simulink model "SingleInverterSim"  (R2020b)
settings: Solver=FixedStepAuto  StartTime=0.0  StopTime=3  FixedStep=Ts  RelTol=1e-3
values from neighbouring files (symbols this model uses):
  Cf = 0.02/W    (= 6.36619772368e-05)    [CalcSwingDroop.m]    (also in SingleInverterSim_Para.m = 0.02; SingleInverterSim_Para_v2.m = 0.02)
  Lc = 0.01/W    (= 3.18309886184e-05)    [CalcSwingDroop.m]    (also in SingleInverterSim_Para.m = 1e-09; SingleInverterSim_Para_v2.m = 0.01)
  Lf = 0.05/W    (= 0.000159154943092)    [CalcSwingDroop.m]    (also in SingleInverterSim_Para.m = 0.05; SingleInverterSim_Para_v2.m = 0.05)
  m = m*Wbase    (= 15.7079632679)    [CalcSwingDroop.m]    (also in SingleInverterSim_Para.m = 0.05; SingleInverterSim_Para_v2.m = 0.05)
  R_rated_GFL = X_rated_GFL/5    (= 0.08)    [SingleInverterSim_Para.m]
  R_rated_GFM = X_rated_GFM/5    (= 0.06)    [SingleInverterSim_Para.m]
  Sbase = 1    [MainAnalysisImpedanceCircuit.m]    (also in SingleInverterSim_Para.m; SingleInverterSim_Para_v2.m)
  Scale_ki_v = 20    [SingleInverterSim_Para.m]    (also in SingleInverterSim_Para_v2.m)
  Ts = 1/Fs    (= 0.0001)    [SingleInverterSim_Para.m]    (also in SingleInverterSim_Para_v2.m)
  Vbase = 1    [MainAnalysisImpedanceCircuit.m]    (also in SingleInverterSim_Para.m; SingleInverterSim_Para_v2.m)
  w_droop = 0.1*2*pi    (= 0.628318530718)    [SingleInverterSim_Para.m]    (also in SingleInverterSim_Para_v2.m = 62.8318530718)
  w_i_GFL = 250 *2*pi    (= 1570.79632679)    [SingleInverterSim_Para.m]    (also in SingleInverterSim_Para_v2.m = 3141.59265359)
  w_i_GFM = 500*2*pi    (= 3141.59265359)    [SingleInverterSim_Para.m]    (also in SingleInverterSim_Para_v2.m)
  w_pll = 15 *2*pi    (= 94.2477796077)    [SingleInverterSim_Para.m]    (also in SingleInverterSim_Para_v2.m = 62.8318530718)
  w_tau = 1e3 *2*pi    (= 6283.18530718)    [SingleInverterSim_Para.m]    (also in SingleInverterSim_Para_v2.m)
  w_v_GFM = 250 *2*pi    (= 1570.79632679)    [SingleInverterSim_Para.m]    (also in SingleInverterSim_Para_v2.m)
  Wbase = 2*pi*50    (= 314.159265359)    [CalcSwingDroop.m]    (also in MainAnalysisImpedanceCircuit.m; SingleInverterSim_Para.m; SingleInverterSim_Para_v2.m)
  X_rated_GFL = 0.4    [SingleInverterSim_Para.m]
  X_rated_GFM = 0.3    [SingleInverterSim_Para.m]
  Zbase = Vbase/Ibase    (= 1)    [MainAnalysisImpedanceCircuit.m]    (also in SingleInverterSim_Para.m; SingleInverterSim_Para_v2.m)
undefined symbols (not defined in the file or in its folder): DiscIntNeverNeededParam, initial, magnitude
libraries: powerlib x230, SimplexPS x57, SimplexPS_2015a x10, SimplusGT x3
(part 2 of 5)

== system SingleInverterSim/AC Infinite Bus (Voltage Type)5 ==
  note: Model for voltage-type infinite bus.
      |
      | Author(s): Yitong Li
  note: Electrical Circuit
  note: Auxiliary
  Bus Creator : BusCreator  Inputs=7
  Constant : Constant  Value=[vd vq]
  Constant1 : Constant  Value=w
  Constant2 : Constant  Value=theta0
  Constant3 : Constant  Value=2*pi
  Demux : Demux  Outputs=3
  Discrete-Time Integrator : DiscreteIntegrator  IntegratorMethod=Integration: Trapezoidal  InitialConditionSource=external  SampleTime=-1  ICPrevOutput=DiscIntNeverNeededParam  ICPrevScaledInput=DiscIntNeverNeededParam
  Gain1 : Gain  Gain=Vbase
  Gain2 : Gain  Gain=1/Wbase
  Gain3 : Gain  Gain=1/(Sbase/Vbase)
  Math Function1 : Math  Operator=mod  SignedPower=on  SaturateOnIntegerOverflow=on
  Mux : Mux  Inputs=3
  PQ Calculation (dq-Frame) : SimplexPS/PQ Calculation (dq-Frame)  SystemSampleTime=-1  VariantActivationTime=update diagram  Latency=0  AutoFrameSizeCalculation=off
      settings: SourceProductName=Simplex Power Systems
  Ra : powerlib/Elements/Series RLC Branch  LConnTagsString=__new0  RConnTagsString=__new0  BranchType=R  Resistance=R  Inductance=1e-3  SetiL0=off  InitialCurrent=0  Capacitance=1e-6  Setx0=off  InitialVoltage=0  Measurements=None
  Rb : powerlib/Elements/Series RLC Branch  LConnTagsString=__new0  RConnTagsString=__new0  BranchType=R  Resistance=R  Inductance=1e-3  SetiL0=off  InitialCurrent=0  Capacitance=1e-6  Setx0=off  InitialVoltage=0  Measurements=None
  Rc : powerlib/Elements/Series RLC Branch  LConnTagsString=__new0  RConnTagsString=__new0  BranchType=R  Resistance=R  Inductance=1e-3  SetiL0=off  InitialCurrent=0  Capacitance=1e-6  Setx0=off  InitialVoltage=0  Measurements=None
  "abc -> dq (Power-Invariant)" : SimplexPS/abc -> dq (Power-Invariant)  SystemSampleTime=-1  VariantActivationTime=update diagram  Latency=0  AutoFrameSizeCalculation=off
      settings: SourceProductName=Simplex Power Systems
  "dq -> abc (Power-Invariant)" : SimplexPS/dq -> abc (Power-Invariant)  SystemSampleTime=-1  VariantActivationTime=update diagram  Latency=0  AutoFrameSizeCalculation=off
      settings: SourceProductName=Simplex Power Systems
  ia : powerlib/Measurements/Current Measurement  PhasorSimulation=off  OutputType=Complex  PSBequivalent=0
  ib : powerlib/Measurements/Current Measurement  PhasorSimulation=off  OutputType=Complex  PSBequivalent=0
  ic : powerlib/Measurements/Current Measurement  PhasorSimulation=off  OutputType=Complex  PSBequivalent=0
  va : powerlib/Electrical Sources/Controlled Voltage Source  Initialize=on  Source_Type=AC  Amplitude=0  Phase=0  Frequency=0  Measurements=None
  vb : powerlib/Electrical Sources/Controlled Voltage Source  Initialize=on  Source_Type=AC  Amplitude=0  Phase=0  Frequency=0  Measurements=None
  vc : powerlib/Electrical Sources/Controlled Voltage Source  Initialize=on  Source_Type=AC  Amplitude=0  Phase=0  Frequency=0  Measurements=None
  a : PMIOPort  Side=Left
  b : PMIOPort  Port=2  Side=Left
  c : PMIOPort  Port=3  Side=Left
  n : PMIOPort  Port=4  Side=Left
  m : Outport
  wires:
  [v_abc] -> Gain1/1
  Demux/1 -> va/1
  Demux/2 -> vb/1
  Demux/3 -> vc/1
  Math Function1/1 -> "dq -> abc (Power-Invariant)"/2, [theta]
  Constant2/1 -> Discrete-Time Integrator/2
  Constant1/1 -> Discrete-Time Integrator/1, [w]
  "dq -> abc (Power-Invariant)"/1 -> [v_abc]
  Constant3/1 -> Math Function1/2
  Constant/1 -> "dq -> abc (Power-Invariant)"/1, [v_dq]
  Discrete-Time Integrator/1 -> Math Function1/1
  [v_dq] -> Bus Creator/1  "v_dq"
  [i_abc] -> Bus Creator/4  "i_abc"
  [w] -> Gain2/1  "w"
  [v_abc] -> Bus Creator/3  "v_abc"
  Gain2/1 -> Bus Creator/5  "w"
  [i_dq] -> Bus Creator/2  "i_dq"
  Bus Creator/1 -> m/1
  [theta] -> Bus Creator/6  "theta"
  ia/1 -> Mux/1
  ib/1 -> Mux/2
  ic/1 -> Mux/3
  [i_abc] -> "abc -> dq (Power-Invariant)"/1
  [theta] -> "abc -> dq (Power-Invariant)"/2
  "abc -> dq (Power-Invariant)"/1 -> [i_dq]
  Gain1/1 -> Demux/1
  Mux/1 -> Gain3/1
  Gain3/1 -> [i_abc]
  [v_dq] -> PQ Calculation (dq-Frame)/1  "v_dq"
  [i_dq] -> PQ Calculation (dq-Frame)/2  "i_dq"
  PQ Calculation (dq-Frame)/1 -> [pq]
  [pq] -> Bus Creator/7  "pq"
  connections:
  vc/LConn1 -- n/RConn1 -- va/LConn1 -- vb/LConn1
  ia/RConn1 -- va/RConn1
  ib/RConn1 -- vb/RConn1
  ic/RConn1 -- vc/RConn1
  Ra/RConn1 -- ia/LConn1
  Ra/LConn1 -- a/RConn1
  ib/LConn1 -- Rb/RConn1
  Rb/LConn1 -- b/RConn1
  Rc/RConn1 -- ic/LConn1
  Rc/LConn1 -- c/RConn1

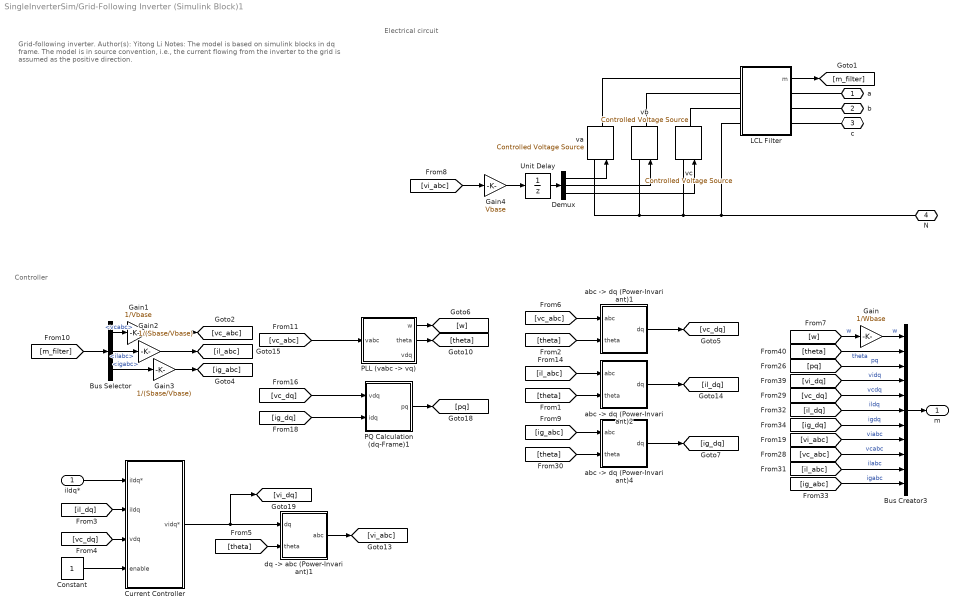
== system SingleInverterSim/Grid-Following Inverter (Simulink Block)1 ==
  note: Grid-following inverter.
      |
      | Author(s): Yitong Li
      |
      | Notes:
      |
      | The model is based on simulink blocks in dq frame.
      |
      | The model is in source convention, i.e., the current flowing from the inverter to the grid is assumed as the positive direction.
  note: Electrical circuit
  note: Controller
  ildq* : Inport
  Bus Creator3 : BusCreator  Inputs=11
  Bus Selector : BusSelector  OutputSignals=vcabc,ilabc,igabc
  Constant : Constant
  Current Controller : Subsystem  mask{Ts=Ts, Wbase=Wbase, Lf=Lf/Wbase, Kg=0, Kp=w_i*Lf/Wbase, Ki=w_i*w_i/4*Lf/Wbase, vdmax=inf, vqmax=inf, Kcd=0}
      mask prompts: Ts "Sampling Time (s)"; Wbase "Base Angular Frequency (rad/s)"; Lf "Inductance"; Kg "Estimator Gain"; Kp "Proportional Gain"; Ki "Integral Gain"; vdmax "Voltage D Limit"; vqmax "Voltage Q Limit"; Kcd "Cross Decoupling Gain"
  Demux : Demux  Outputs=3
  Gain : Gain  Gain=1/Wbase
  Gain1 : Gain  Gain=1/Vbase
  Gain2 : Gain  Gain=1/(Sbase/Vbase)
  Gain3 : Gain  Gain=1/(Sbase/Vbase)
  Gain4 : Gain  Gain=Vbase
  LCL Filter : Subsystem  AncestorBlock=SimplexPS/LCL Filter  mask{Lf=Lf*(Vbase^2/Sbase)/Wbase, Rf=Lf*(Vbase^2/Sbase)/5, Lc=Lc*(Vbase^2/Sbase)/Wbase, Rc=Lc*(Vbase^2/Sbase)/5, Cf=Cf*(Sbase/Vbase^2)/Wbase, Rd=1e-5*(Vbase^2/Sbase)}
      mask prompts: Lf "Lf (H)"; Rf "Rf (Ohm)"; Lc "Lc (H)"; Rc "Rc (Ohm)"; Cf "Cf (F)"; Rd "Rd (Ohm)"
  "PLL (vabc -> vq)" : Subsystem  AncestorBlock=|  mask{Ts=Ts, Vbase=Vbase, Wbase=Wbase, w_pll=w_pll, w_tau=w_tau, theta0=0}
      | SimplusGT/PLL
      | (vabc -> vq)
      mask prompts: Ts "Ts (s), sampling period"; Vbase "Vbase (V), base voltage"; Wbase "Wbase (rad/s), base angular frequency"; w_pll "w_pll (rad/s), PLL bandwidth"; w_tau "w_tau (rad/s), low-pass filter bandwidth"; theta0 "theta0 (rad), initial angle"
  PQ Calculation (dq-Frame)1 : Subsystem  AncestorBlock=|
      | SimplusGT/PQ Calculation
      | (dq-Frame)
  Unit Delay : UnitDelay  SampleTime=-1  HasFrameUpgradeWarning=on
  "abc -> dq (Power-Invariant)1" : Subsystem  AncestorBlock=|
      | SimplusGT/abc -> dq
      | (Power-Invariant)
  "abc -> dq (Power-Invariant)2" : Subsystem  AncestorBlock=|
      | SimplusGT/abc -> dq
      | (Power-Invariant)
  "abc -> dq (Power-Invariant)4" : Subsystem  AncestorBlock=|
      | SimplusGT/abc -> dq
      | (Power-Invariant)
  "dq -> abc (Power-Invariant)1" : Subsystem  AncestorBlock=|
      | SimplusGT/dq -> abc
      | (Power-Invariant)
  va : powerlib/Electrical Sources/Controlled Voltage Source  Initialize=on  Source_Type=AC  Amplitude=0  Phase=0  Frequency=0  Measurements=None
  vb : powerlib/Electrical Sources/Controlled Voltage Source  Initialize=on  Source_Type=AC  Amplitude=0  Phase=0  Frequency=0  Measurements=None
  vc : powerlib/Electrical Sources/Controlled Voltage Source  Initialize=on  Source_Type=AC  Amplitude=0  Phase=0  Frequency=0  Measurements=None
  a : PMIOPort  Side=Right
  b : PMIOPort  Port=2  Side=Right
  c : PMIOPort  Port=3  Side=Right
  N : PMIOPort  Port=4  Side=Right
  m : Outport
  wires:
  [vi_abc] -> Gain4/1
  Gain4/1 -> Unit Delay/1
  Gain3/1 -> [ig_abc]
  Gain2/1 -> [il_abc]
  Gain1/1 -> [vc_abc]
  [ig_abc] -> Bus Creator3/11  "igabc"
  [il_abc] -> Bus Creator3/10  "ilabc"
  [vc_abc] -> Bus Creator3/9  "vcabc"
  [vi_abc] -> Bus Creator3/8  "viabc"
  [ig_dq] -> Bus Creator3/7  "igdq"
  [il_dq] -> Bus Creator3/6  "ildq"
  [vc_dq] -> Bus Creator3/5  "vcdq"
  [vi_dq] -> Bus Creator3/4  "vidq"
  [pq] -> Bus Creator3/3  "pq"
  [theta] -> Bus Creator3/2  "theta"
  Gain/1 -> Bus Creator3/1  "w"
  [w] -> Gain/1  "w"
  Bus Selector/1 -> Gain1/1  "<vcabc>"
  Unit Delay/1 -> Demux/1
  [m_filter] -> Bus Selector/1
  "abc -> dq (Power-Invariant)2"/1(dq) -> [il_dq]
  "abc -> dq (Power-Invariant)4"/1(dq) -> [ig_dq]
  "abc -> dq (Power-Invariant)1"/1(dq) -> [vc_dq]
  [vc_abc] -> "PLL (vabc -> vq)"/1(vabc)
  [il_dq] -> Current Controller/2(iIdq)
  ildq*/1 -> Current Controller/1(iIdq*)
  [ig_dq] -> PQ Calculation (dq-Frame)1/2(idq)
  PQ Calculation (dq-Frame)1/1(pq) -> [pq]
  [vc_dq] -> PQ Calculation (dq-Frame)1/1(vdq)
  [theta] -> "dq -> abc (Power-Invariant)1"/2(theta)
  Current Controller/1(vidq*) -> [vi_dq], "dq -> abc (Power-Invariant)1"/1(dq)
  [vc_dq] -> Current Controller/3(vdq)
  Constant/1 -> Current Controller/4(enable)
  "PLL (vabc -> vq)"/1(w) -> [w]
  "PLL (vabc -> vq)"/2(theta) -> [theta]
  Bus Selector/2 -> Gain2/1  "<ilabc>"
  Bus Selector/3 -> Gain3/1  "<igabc>"
  [theta] -> "abc -> dq (Power-Invariant)4"/2(theta)
  [ig_abc] -> "abc -> dq (Power-Invariant)4"/1(abc)
  [il_abc] -> "abc -> dq (Power-Invariant)2"/1(abc)
  [vc_abc] -> "abc -> dq (Power-Invariant)1"/1(abc)
  [theta] -> "abc -> dq (Power-Invariant)2"/2(theta)
  [theta] -> "abc -> dq (Power-Invariant)1"/2(theta)
  Demux/3 -> vc/1
  Demux/2 -> vb/1
  Demux/1 -> va/1
  LCL Filter/1(m) -> [m_filter]
  Bus Creator3/1 -> m/1
  "dq -> abc (Power-Invariant)1"/1(abc) -> [vi_abc]
  connections:
  LCL Filter/LConn3 -- vc/RConn1
  va/LConn1 -- vb/LConn1 -- vc/LConn1 -- LCL Filter/LConn4 -- N/RConn1
  LCL Filter/RConn3 -- c/RConn1
  LCL Filter/RConn2 -- b/RConn1
  LCL Filter/RConn1 -- a/RConn1
  LCL Filter/LConn1 -- va/RConn1
  LCL Filter/LConn2 -- vb/RConn1

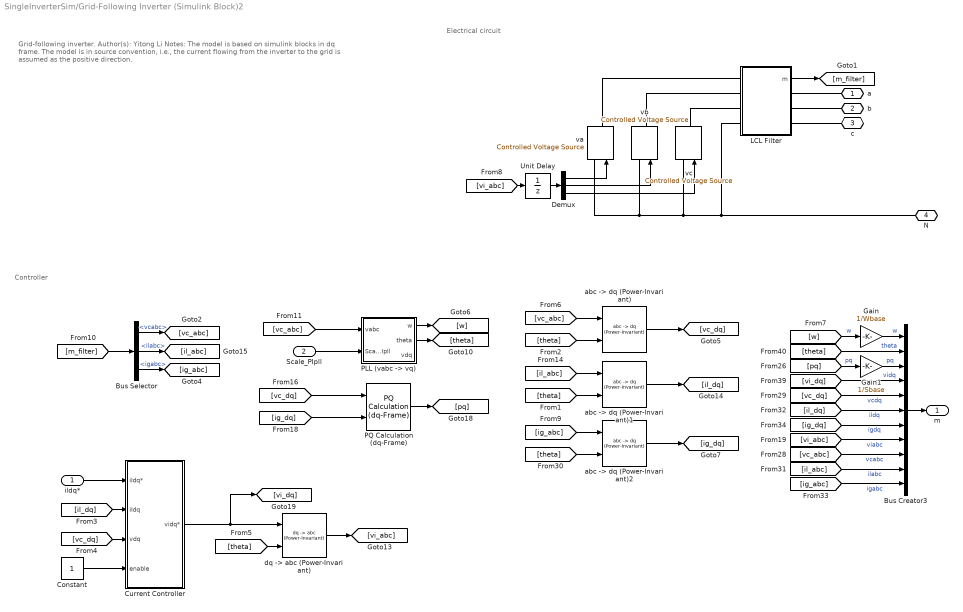
== system SingleInverterSim/Grid-Following Inverter (Simulink Block)2 ==
  note: Controller
  note: Electrical circuit
  note: Grid-following inverter.
      |
      | Author(s): Yitong Li
      |
      | Notes:
      |
      | The model is based on simulink blocks in dq frame.
      |
      | The model is in source convention, i.e., the current flowing from the inverter to the grid is assumed as the positive direction.
  ildq* : Inport
  Scale_PIpll : Inport  Port=2
  Bus Creator3 : BusCreator  Inputs=11
  Bus Selector : BusSelector  OutputSignals=vcabc,ilabc,igabc
  Constant : Constant
  Current Controller : Subsystem  mask{Ts=Ts, Wbase=Wbase, Lf=Lf*(Vbase^2/Sbase)/Wbase, Kg=0, Kp=w_i*Lf*(Vbase^2/Sbase)/Wbase, Ki=w_i*w_i/4*Lf*(Vbase^2/Sbase)/Wbase, vdmax=inf, vqmax=inf, Kcd=0}
      mask prompts: Ts "Sampling Time (s)"; Wbase "Base Angular Frequency (rad/s)"; Lf "Inductance"; Kg "Estimator Gain"; Kp "Proportional Gain"; Ki "Integral Gain"; vdmax "Voltage D Limit"; vqmax "Voltage Q Limit"; Kcd "Cross Decoupling Gain"
  Demux : Demux  Outputs=3
  Gain : Gain  Gain=1/Wbase
  Gain1 : Gain  Gain=1/Sbase
  LCL Filter : Subsystem  AncestorBlock=SimplexPS/LCL Filter  mask{Lf=Lf*Zbase/Wbase, Rf=Lf/5, Lc=Lc*(Vbase^2/Sbase)/Wbase, Rc=Lc/5, Cf=Cf*(Sbase/Vbase^2)/Wbase, Rd=1e-20}
      mask prompts: Lf "Lf (H)"; Rf "Rf (Ohm)"; Lc "Lc (H)"; Rc "Rc (Ohm)"; Cf "Cf (F)"; Rd "Rd (Ohm)"
  "PLL (vabc -> vq)" : Subsystem  AncestorBlock=|  mask{Ts=Ts, Vbase=Vbase, Wbase=Wbase, w_pll=w_pll, w_tau=w_tau, theta0=0}
      | SimplexPS/PLL
      | (vabc -> vq)
      mask prompts: Ts "Ts (s), sampling period"; Vbase "Vbase (V), base voltage"; Wbase "Wbase (rad/s), base angular frequency"; w_pll "w_pll (rad/s), PLL bandwidth"; w_tau "w_tau (rad/s), low-pass filter bandwidth"; theta0 "theta0 (rad), initial angle"
  PQ Calculation (dq-Frame) : SimplexPS/PQ Calculation (dq-Frame)  SystemSampleTime=-1  VariantActivationTime=update diagram  Latency=0  AutoFrameSizeCalculation=off
      settings: SourceProductName=Simplex Power Systems
  Unit Delay : UnitDelay  SampleTime=-1  HasFrameUpgradeWarning=on
  "abc -> dq (Power-Invariant)" : SimplexPS/abc -> dq (Power-Invariant)  SystemSampleTime=-1  VariantActivationTime=update diagram  Latency=0  AutoFrameSizeCalculation=off
      settings: SourceProductName=Simplex Power Systems
  "abc -> dq (Power-Invariant)1" : SimplexPS/abc -> dq (Power-Invariant)  SystemSampleTime=-1  VariantActivationTime=update diagram  Latency=0  AutoFrameSizeCalculation=off
      settings: SourceProductName=Simplex Power Systems
  "abc -> dq (Power-Invariant)2" : SimplexPS/abc -> dq (Power-Invariant)  SystemSampleTime=-1  VariantActivationTime=update diagram  Latency=0  AutoFrameSizeCalculation=off
      settings: SourceProductName=Simplex Power Systems
  "dq -> abc (Power-Invariant)" : SimplexPS/dq -> abc (Power-Invariant)  SystemSampleTime=-1  VariantActivationTime=update diagram  Latency=0  AutoFrameSizeCalculation=off
      settings: SourceProductName=Simplex Power Systems
  va : powerlib/Electrical Sources/Controlled Voltage Source  Initialize=on  Source_Type=AC  Amplitude=0  Phase=0  Frequency=0  Measurements=None
  vb : powerlib/Electrical Sources/Controlled Voltage Source  Initialize=on  Source_Type=AC  Amplitude=0  Phase=0  Frequency=0  Measurements=None
  vc : powerlib/Electrical Sources/Controlled Voltage Source  Initialize=on  Source_Type=AC  Amplitude=0  Phase=0  Frequency=0  Measurements=None
  a : PMIOPort  Side=Right
  b : PMIOPort  Port=2  Side=Right
  c : PMIOPort  Port=3  Side=Right
  N : PMIOPort  Port=4  Side=Right
  m : Outport
  wires:
  "dq -> abc (Power-Invariant)"/1 -> [vi_abc]
  Bus Creator3/1 -> m/1
  LCL Filter/1(m) -> [m_filter]
  Demux/1 -> va/1
  Demux/2 -> vb/1
  Demux/3 -> vc/1
  [theta] -> "abc -> dq (Power-Invariant)"/2
  [theta] -> "abc -> dq (Power-Invariant)1"/2
  [vc_abc] -> "abc -> dq (Power-Invariant)"/1
  [il_abc] -> "abc -> dq (Power-Invariant)1"/1
  [ig_abc] -> "abc -> dq (Power-Invariant)2"/1
  [theta] -> "abc -> dq (Power-Invariant)2"/2
  Bus Selector/3 -> [ig_abc]  "<igabc>"
  Bus Selector/2 -> [il_abc]  "<ilabc>"
  "PLL (vabc -> vq)"/2(theta) -> [theta]
  "PLL (vabc -> vq)"/1(w) -> [w]
  Constant/1 -> Current Controller/4(enable)
  [vc_dq] -> Current Controller/3(vdq)
  Current Controller/1(vidq*) -> [vi_dq], "dq -> abc (Power-Invariant)"/1
  [theta] -> "dq -> abc (Power-Invariant)"/2
  [vc_dq] -> PQ Calculation (dq-Frame)/1
  PQ Calculation (dq-Frame)/1 -> [pq]
  [ig_dq] -> PQ Calculation (dq-Frame)/2
  ildq*/1 -> Current Controller/1(iIdq*)
  [il_dq] -> Current Controller/2(iIdq)
  [vc_abc] -> "PLL (vabc -> vq)"/1(vabc)
  "abc -> dq (Power-Invariant)"/1 -> [vc_dq]
  "abc -> dq (Power-Invariant)2"/1 -> [ig_dq]
  "abc -> dq (Power-Invariant)1"/1 -> [il_dq]
  [m_filter] -> Bus Selector/1
  [vi_abc] -> Unit Delay/1
  Unit Delay/1 -> Demux/1
  Bus Selector/1 -> [vc_abc]  "<vcabc>"
  [w] -> Gain/1  "w"
  [pq] -> Gain1/1  "pq"
  Gain/1 -> Bus Creator3/1  "w"
  [theta] -> Bus Creator3/2  "theta"
  Gain1/1 -> Bus Creator3/3  "pq"
  [vi_dq] -> Bus Creator3/4  "vidq"
  [vc_dq] -> Bus Creator3/5  "vcdq"
  [il_dq] -> Bus Creator3/6  "ildq"
  [ig_dq] -> Bus Creator3/7  "igdq"
  [vi_abc] -> Bus Creator3/8  "viabc"
  [vc_abc] -> Bus Creator3/9  "vcabc"
  [il_abc] -> Bus Creator3/10  "ilabc"
  [ig_abc] -> Bus Creator3/11  "igabc"
  Scale_PIpll/1 -> "PLL (vabc -> vq)"/2(Scale_PIpll)
  connections:
  LCL Filter/LConn2 -- vb/RConn1
  LCL Filter/LConn1 -- va/RConn1
  LCL Filter/RConn1 -- a/RConn1
  LCL Filter/RConn2 -- b/RConn1
  LCL Filter/RConn3 -- c/RConn1
  N/RConn1 -- LCL Filter/LConn4 -- vc/LConn1 -- vb/LConn1 -- va/LConn1
  LCL Filter/LConn3 -- vc/RConn1

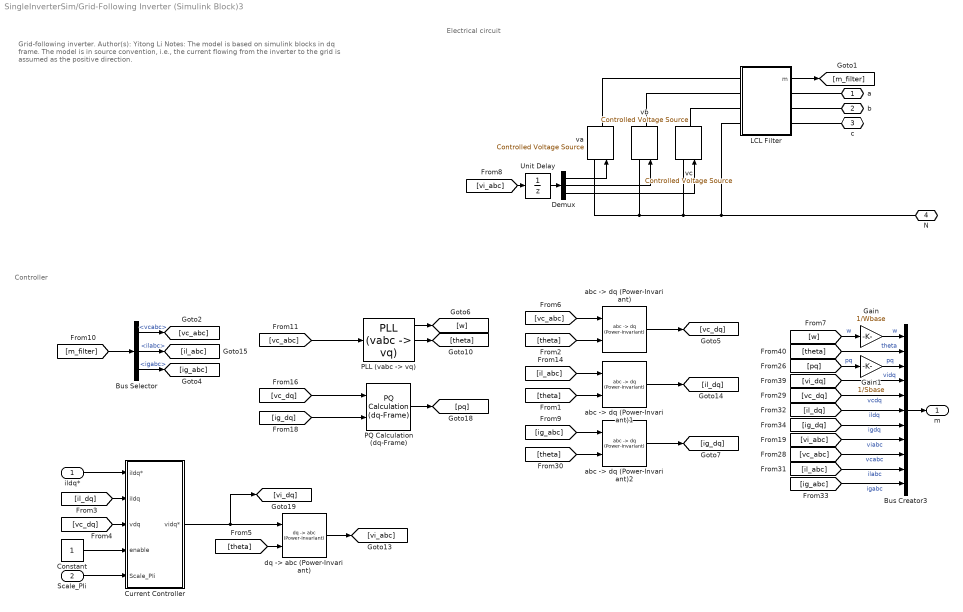
== system SingleInverterSim/Grid-Following Inverter (Simulink Block)3 ==
  note: Controller
  note: Electrical circuit
  note: Grid-following inverter.
      |
      | Author(s): Yitong Li
      |
      | Notes:
      |
      | The model is based on simulink blocks in dq frame.
      |
      | The model is in source convention, i.e., the current flowing from the inverter to the grid is assumed as the positive direction.
  ildq* : Inport
  Scale_PIi : Inport  Port=2
  Bus Creator3 : BusCreator  Inputs=11
  Bus Selector : BusSelector  OutputSignals=vcabc,ilabc,igabc
  Constant : Constant
  Current Controller : Subsystem  mask{Ts=Ts, Wbase=Wbase, Lf=Lf*(Vbase^2/Sbase)/Wbase, Kg=0, Kp=w_i*Lf*(Vbase^2/Sbase)/Wbase, Ki=w_i*w_i/4*Lf*(Vbase^2/Sbase)/Wbase, vdmax=inf, vqmax=inf, Kcd=0}
      mask prompts: Ts "Sampling Time (s)"; Wbase "Base Angular Frequency (rad/s)"; Lf "Inductance"; Kg "Estimator Gain"; Kp "Proportional Gain"; Ki "Integral Gain"; vdmax "Voltage D Limit"; vqmax "Voltage Q Limit"; Kcd "Cross Decoupling Gain"
  Demux : Demux  Outputs=3
  Gain : Gain  Gain=1/Wbase
  Gain1 : Gain  Gain=1/Sbase
  LCL Filter : Subsystem  AncestorBlock=SimplexPS/LCL Filter  mask{Lf=Lf*Zbase/Wbase, Rf=Lf/5, Lc=Lc*(Vbase^2/Sbase)/Wbase, Rc=Lc/5, Cf=Cf*(Sbase/Vbase^2)/Wbase, Rd=1e-20}
      mask prompts: Lf "Lf (H)"; Rf "Rf (Ohm)"; Lc "Lc (H)"; Rc "Rc (Ohm)"; Cf "Cf (F)"; Rd "Rd (Ohm)"
  "PLL (vabc -> vq)" : SimplexPS/PLL (vabc -> vq)  Ts=Ts  Vbase=Vbase  Wbase=Wbase  w_pll=w_pll  w_tau=w_tau  theta0=0
      settings: SourceProductName=Simplex Power Systems
  PQ Calculation (dq-Frame) : SimplexPS/PQ Calculation (dq-Frame)  SystemSampleTime=-1  VariantActivationTime=update diagram  Latency=0  AutoFrameSizeCalculation=off
      settings: SourceProductName=Simplex Power Systems
  Unit Delay : UnitDelay  SampleTime=-1  HasFrameUpgradeWarning=on
  "abc -> dq (Power-Invariant)" : SimplexPS/abc -> dq (Power-Invariant)  SystemSampleTime=-1  VariantActivationTime=update diagram  Latency=0  AutoFrameSizeCalculation=off
      settings: SourceProductName=Simplex Power Systems
  "abc -> dq (Power-Invariant)1" : SimplexPS/abc -> dq (Power-Invariant)  SystemSampleTime=-1  VariantActivationTime=update diagram  Latency=0  AutoFrameSizeCalculation=off
      settings: SourceProductName=Simplex Power Systems
  "abc -> dq (Power-Invariant)2" : SimplexPS/abc -> dq (Power-Invariant)  SystemSampleTime=-1  VariantActivationTime=update diagram  Latency=0  AutoFrameSizeCalculation=off
      settings: SourceProductName=Simplex Power Systems
  "dq -> abc (Power-Invariant)" : SimplexPS/dq -> abc (Power-Invariant)  SystemSampleTime=-1  VariantActivationTime=update diagram  Latency=0  AutoFrameSizeCalculation=off
      settings: SourceProductName=Simplex Power Systems
  va : powerlib/Electrical Sources/Controlled Voltage Source  Initialize=on  Source_Type=AC  Amplitude=0  Phase=0  Frequency=0  Measurements=None
  vb : powerlib/Electrical Sources/Controlled Voltage Source  Initialize=on  Source_Type=AC  Amplitude=0  Phase=0  Frequency=0  Measurements=None
  vc : powerlib/Electrical Sources/Controlled Voltage Source  Initialize=on  Source_Type=AC  Amplitude=0  Phase=0  Frequency=0  Measurements=None
  a : PMIOPort  Side=Right
  b : PMIOPort  Port=2  Side=Right
  c : PMIOPort  Port=3  Side=Right
  N : PMIOPort  Port=4  Side=Right
  m : Outport
  wires:
  "dq -> abc (Power-Invariant)"/1 -> [vi_abc]
  Bus Creator3/1 -> m/1
  LCL Filter/1(m) -> [m_filter]
  Demux/1 -> va/1
  Demux/2 -> vb/1
  Demux/3 -> vc/1
  [theta] -> "abc -> dq (Power-Invariant)"/2
  [theta] -> "abc -> dq (Power-Invariant)1"/2
  [vc_abc] -> "abc -> dq (Power-Invariant)"/1
  [il_abc] -> "abc -> dq (Power-Invariant)1"/1
  [ig_abc] -> "abc -> dq (Power-Invariant)2"/1
  [theta] -> "abc -> dq (Power-Invariant)2"/2
  Bus Selector/3 -> [ig_abc]  "<igabc>"
  Bus Selector/2 -> [il_abc]  "<ilabc>"
  "PLL (vabc -> vq)"/2 -> [theta]
  "PLL (vabc -> vq)"/1 -> [w]
  Constant/1 -> Current Controller/4(enable)
  [vc_dq] -> Current Controller/3(vdq)
  Current Controller/1(vidq*) -> [vi_dq], "dq -> abc (Power-Invariant)"/1
  [theta] -> "dq -> abc (Power-Invariant)"/2
  [vc_dq] -> PQ Calculation (dq-Frame)/1
  PQ Calculation (dq-Frame)/1 -> [pq]
  [ig_dq] -> PQ Calculation (dq-Frame)/2
  ildq*/1 -> Current Controller/1(iIdq*)
  [il_dq] -> Current Controller/2(iIdq)
  [vc_abc] -> "PLL (vabc -> vq)"/1
  "abc -> dq (Power-Invariant)"/1 -> [vc_dq]
  "abc -> dq (Power-Invariant)2"/1 -> [ig_dq]
  "abc -> dq (Power-Invariant)1"/1 -> [il_dq]
  [m_filter] -> Bus Selector/1
  [vi_abc] -> Unit Delay/1
  Unit Delay/1 -> Demux/1
  Bus Selector/1 -> [vc_abc]  "<vcabc>"
  [w] -> Gain/1  "w"
  [pq] -> Gain1/1  "pq"
  Gain/1 -> Bus Creator3/1  "w"
  [theta] -> Bus Creator3/2  "theta"
  Gain1/1 -> Bus Creator3/3  "pq"
  [vi_dq] -> Bus Creator3/4  "vidq"
  [vc_dq] -> Bus Creator3/5  "vcdq"
  [il_dq] -> Bus Creator3/6  "ildq"
  [ig_dq] -> Bus Creator3/7  "igdq"
  [vi_abc] -> Bus Creator3/8  "viabc"
  [vc_abc] -> Bus Creator3/9  "vcabc"
  [il_abc] -> Bus Creator3/10  "ilabc"
  [ig_abc] -> Bus Creator3/11  "igabc"
  Scale_PIi/1 -> Current Controller/5(Scale_PIi)
  connections:
  LCL Filter/LConn2 -- vb/RConn1
  LCL Filter/LConn1 -- va/RConn1
  LCL Filter/RConn1 -- a/RConn1
  LCL Filter/RConn2 -- b/RConn1
  LCL Filter/RConn3 -- c/RConn1
  N/RConn1 -- LCL Filter/LConn4 -- vc/LConn1 -- vb/LConn1 -- va/LConn1
  LCL Filter/LConn3 -- vc/RConn1

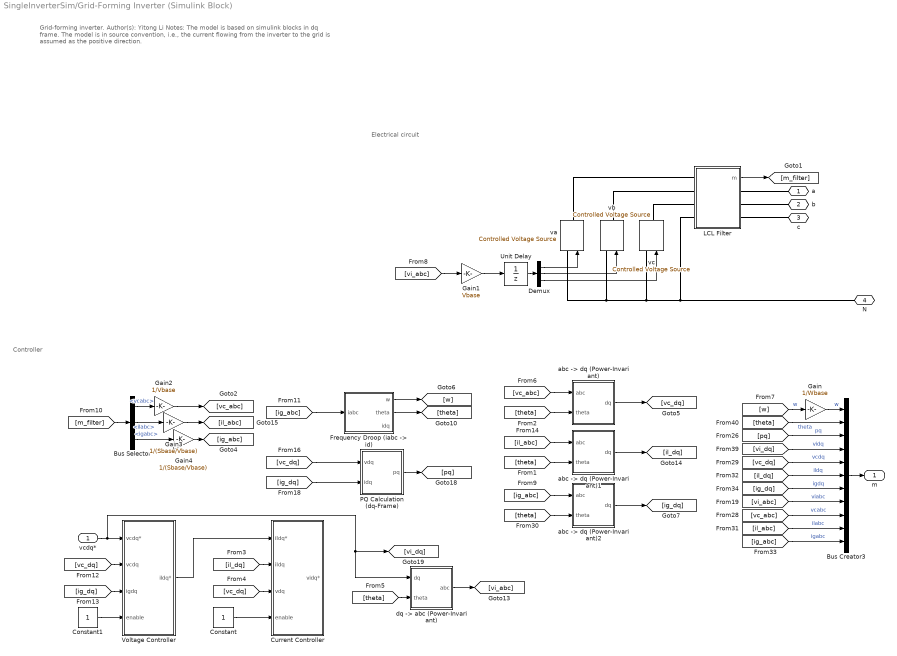
== system SingleInverterSim/Grid-Forming Inverter (Simulink Block) ==
  note: Grid-forming inverter.
      |
      | Author(s): Yitong Li
      |
      | Notes:
      |
      | The model is based on simulink blocks in dq frame.
      |
      | The model is in source convention, i.e., the current flowing from the inverter to the grid is assumed as the positive direction.
  note: Electrical circuit
  note: Controller
  vcdq* : Inport
  Bus Creator3 : BusCreator  Inputs=11
  Bus Selector : BusSelector  OutputSignals=vcabc,ilabc,igabc
  Constant : Constant
  Constant1 : Constant
  Current Controller : Subsystem  mask{Ts=Ts, Wbase=Wbase, Lf=Lf/Wbase, Kg=0, Kp=w_i*Lf/Wbase, Ki=w_i*w_i/4*Lf/Wbase, xdmax=inf, xqmax=inf, Kcd=0}
      mask prompts: Ts "Sampling Time (s)"; Wbase "Base Angular Frequency (rad/s)"; Lf "Inductance"; Kg "Estimator Gain"; Kp "Proportional Gain"; Ki "Integral Gain"; xdmax "Voltage D Limit"; xqmax "Voltage Q Limit"; Kcd "Cross Decoupling Gain"
  Demux : Demux  Outputs=3
  "Frequency Droop (iabc -> id)" : Subsystem  AncestorBlock=|  mask{Ts=Ts, Sbase=Sbase, Vbase=Vbase, Wbase=Wbase, m=m, w_tau=w_droop, theta0=0, i0=0, w0=1}
      | SimplusGT/Frequency Droop
      | (iabc -> id)
      mask prompts: Ts "Ts (s), samping period"; Sbase "Sbase (VA), base power"; Vbase "Vbase (V), base voltage"; Wbase "Wbase (rad/s), base angular frequency"; m "m (pu), droop gain"; w_tau "w_tau (rad/s), low-pass filter bandwidth"; theta0 "theta0 (rad), initial angle"; i0 "i0 (pu), current setting point"; w0 "w0 (pu), frequency setting point"
  Gain : Gain  Gain=1/Wbase
  Gain1 : Gain  Gain=Vbase
  Gain2 : Gain  Gain=1/Vbase
  Gain3 : Gain  Gain=1/(Sbase/Vbase)
  Gain4 : Gain  Gain=1/(Sbase/Vbase)
  LCL Filter : Subsystem  AncestorBlock=SimplexPS/LCL Filter  mask{Lf=Lf*(Vbase^2/Sbase)/Wbase, Rf=Lf*(Vbase^2/Sbase)/5, Lc=Lc*(Vbase^2/Sbase)/Wbase, Rc=Lc*(Vbase^2/Sbase)/5, Cf=Cf*(Sbase/Vbase^2)/Wbase, Rd=1e-5*(Vbase^2/Sbase)}
      mask prompts: Lf "Lf (H)"; Rf "Rf (Ohm)"; Lc "Lc (H)"; Rc "Rc (Ohm)"; Cf "Cf (F)"; Rd "Rd (Ohm)"
  PQ Calculation (dq-Frame) : Subsystem  AncestorBlock=|
      | SimplusGT/PQ Calculation
      | (dq-Frame)
  Unit Delay : UnitDelay  SampleTime=-1  HasFrameUpgradeWarning=on
  Voltage Controller : Subsystem  mask{Ts=Ts, Wbase=Wbase, Cf=Cf/Wbase, Kg=0, Kp=w_v*Cf/Wbase, Ki=w_v*w_v/4*Cf/Wbase*100, xdmax=inf, xqmax=inf, Kcd=0}
      mask prompts: Ts "Sampling Time (s)"; Wbase "Base Angular Frequency (rad/s)"; Cf "Capacitance"; Kg "Estimator Gain"; Kp "Proportional Gain"; Ki "Integral Gain"; xdmax "Current D Limit"; xqmax "Current Q Limit"; Kcd "Cross Decoupling Gain"
  "abc -> dq (Power-Invariant)" : Subsystem  AncestorBlock=|
      | SimplusGT/abc -> dq
      | (Power-Invariant)
  "abc -> dq (Power-Invariant)1" : Subsystem  AncestorBlock=|
      | SimplusGT/abc -> dq
      | (Power-Invariant)
  "abc -> dq (Power-Invariant)2" : Subsystem  AncestorBlock=|
      | SimplusGT/abc -> dq
      | (Power-Invariant)
  "dq -> abc (Power-Invariant)" : Subsystem  AncestorBlock=|
      | SimplusGT/dq -> abc
      | (Power-Invariant)
  va : powerlib/Electrical Sources/Controlled Voltage Source  Initialize=on  Source_Type=AC  Amplitude=0  Phase=0  Frequency=0  Measurements=None
  vb : powerlib/Electrical Sources/Controlled Voltage Source  Initialize=on  Source_Type=AC  Amplitude=0  Phase=0  Frequency=0  Measurements=None
  vc : powerlib/Electrical Sources/Controlled Voltage Source  Initialize=on  Source_Type=AC  Amplitude=0  Phase=0  Frequency=0  Measurements=None
  a : PMIOPort  Side=Right
  b : PMIOPort  Port=2  Side=Right
  c : PMIOPort  Port=3  Side=Right
  N : PMIOPort  Port=4  Side=Right
  m : Outport
  wires:
  Gain1/1 -> Unit Delay/1
  [vi_abc] -> Gain1/1
  Gain4/1 -> [ig_abc]
  Gain3/1 -> [il_abc]
  Gain2/1 -> [vc_abc]
  [ig_dq] -> Voltage Controller/3(igdq)
  [vc_dq] -> Voltage Controller/2(vcdq)
  Constant1/1 -> Voltage Controller/4(enable)
  Voltage Controller/1(ildq*) -> Current Controller/1(iIdq*)
  vcdq*/1 -> [vi_dq], "dq -> abc (Power-Invariant)"/1(dq), Voltage Controller/1(vcdq*)
  [ig_abc] -> Bus Creator3/11  "igabc"
  [il_abc] -> Bus Creator3/10  "ilabc"
  [vc_abc] -> Bus Creator3/9  "vcabc"
  [vi_abc] -> Bus Creator3/8  "viabc"
  [ig_dq] -> Bus Creator3/7  "igdq"
  [il_dq] -> Bus Creator3/6  "ildq"
  [vc_dq] -> Bus Creator3/5  "vcdq"
  [vi_dq] -> Bus Creator3/4  "vidq"
  [pq] -> Bus Creator3/3  "pq"
  [theta] -> Bus Creator3/2  "theta"
  Gain/1 -> Bus Creator3/1  "w"
  [w] -> Gain/1  "w"
  Bus Selector/1 -> Gain2/1  "<vcabc>"
  Unit Delay/1 -> Demux/1
  [m_filter] -> Bus Selector/1
  "abc -> dq (Power-Invariant)1"/1(dq) -> [il_dq]
  "abc -> dq (Power-Invariant)2"/1(dq) -> [ig_dq]
  "abc -> dq (Power-Invariant)"/1(dq) -> [vc_dq]
  [ig_abc] -> "Frequency Droop (iabc -> id)"/1(iabc)
  [il_dq] -> Current Controller/2(iIdq)
  [ig_dq] -> PQ Calculation (dq-Frame)/2(idq)
  PQ Calculation (dq-Frame)/1(pq) -> [pq]
  [vc_dq] -> PQ Calculation (dq-Frame)/1(vdq)
  [theta] -> "dq -> abc (Power-Invariant)"/2(theta)
  [vc_dq] -> Current Controller/3(vdq)
  Constant/1 -> Current Controller/4(enable)
  Bus Selector/2 -> Gain3/1  "<ilabc>"
  Bus Selector/3 -> Gain4/1  "<igabc>"
  [theta] -> "abc -> dq (Power-Invariant)2"/2(theta)
  [ig_abc] -> "abc -> dq (Power-Invariant)2"/1(abc)
  [il_abc] -> "abc -> dq (Power-Invariant)1"/1(abc)
  [vc_abc] -> "abc -> dq (Power-Invariant)"/1(abc)
  [theta] -> "abc -> dq (Power-Invariant)1"/2(theta)
  [theta] -> "abc -> dq (Power-Invariant)"/2(theta)
  Demux/3 -> vc/1
  Demux/2 -> vb/1
  Demux/1 -> va/1
  LCL Filter/1(m) -> [m_filter]
  Bus Creator3/1 -> m/1
  "dq -> abc (Power-Invariant)"/1(abc) -> [vi_abc]
  "Frequency Droop (iabc -> id)"/1(w) -> [w]
  "Frequency Droop (iabc -> id)"/2(theta) -> [theta]
  connections:
  LCL Filter/LConn3 -- vc/RConn1
  va/LConn1 -- vb/LConn1 -- vc/LConn1 -- LCL Filter/LConn4 -- N/RConn1
  LCL Filter/RConn3 -- c/RConn1
  LCL Filter/RConn2 -- b/RConn1
  LCL Filter/RConn1 -- a/RConn1
  LCL Filter/LConn1 -- va/RConn1
  LCL Filter/LConn2 -- vb/RConn1

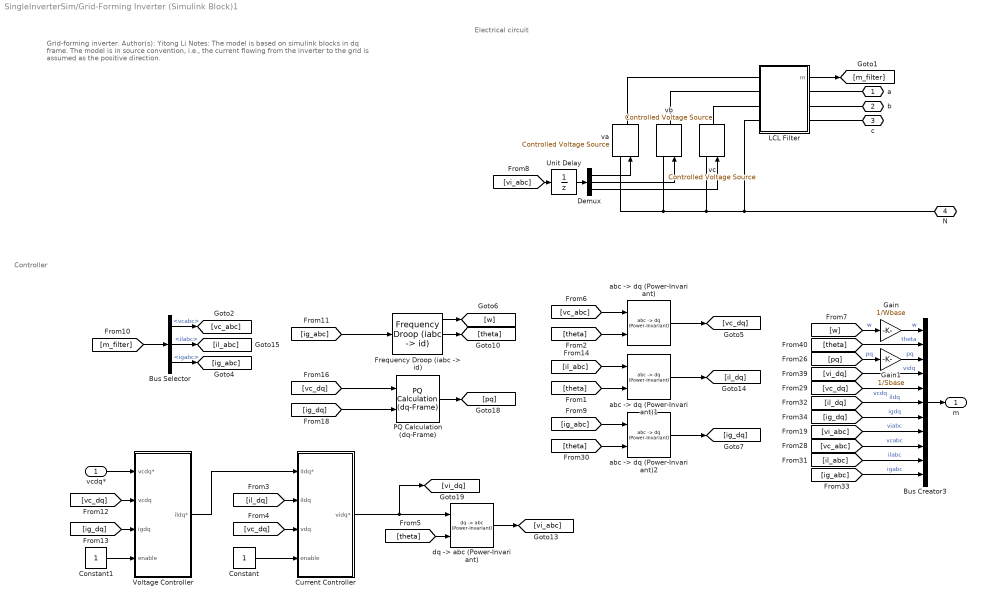
== system SingleInverterSim/Grid-Forming Inverter (Simulink Block)1 ==
  note: Grid-forming inverter.
      |
      | Author(s): Yitong Li
      |
      | Notes:
      |
      | The model is based on simulink blocks in dq frame.
      |
      | The model is in source convention, i.e., the current flowing from the inverter to the grid is assumed as the positive direction.
  note: Electrical circuit
  note: Controller
  vcdq* : Inport
  Bus Creator3 : BusCreator  Inputs=11
  Bus Selector : BusSelector  OutputSignals=vcabc,ilabc,igabc
  Constant : Constant
  Constant1 : Constant
  Current Controller : Subsystem  mask{Ts=Ts, Wbase=Wbase, Lf=Lf*(Vbase^2/Sbase)/Wbase, Kg=0, Kp=w_i*Lf*(Vbase^2/Sbase)/Wbase, Ki=w_i*w_i/4*Lf*(Vbase^2/Sbase)/Wbase, xdmax=inf, xqmax=inf, Kcd=0}
      mask prompts: Ts "Sampling Time (s)"; Wbase "Base Angular Frequency (rad/s)"; Lf "Inductance"; Kg "Estimator Gain"; Kp "Proportional Gain"; Ki "Integral Gain"; xdmax "Voltage D Limit"; xqmax "Voltage Q Limit"; Kcd "Cross Decoupling Gain"
  Demux : Demux  Outputs=3
  "Frequency Droop (iabc -> id)" : SimplexPS/Frequency Droop (iabc -> id)  Ts=Ts  Sbase=Sbase  Vbase=Vbase  Wbase=Wbase  m=m  w_tau=w_droop  theta0=0  i0=0  w0=1
  Gain : Gain  Gain=1/Wbase
  Gain1 : Gain  Gain=1/Sbase
  LCL Filter : Subsystem  AncestorBlock=SimplexPS/LCL Filter  mask{Lf=Lf*(Vbase^2/Sbase)/Wbase, Rf=Lf/10, Lc=Lc*(Vbase^2/Sbase)/Wbase, Rc=1e-20, Cf=Cf*(Sbase/Vbase^2)/Wbase, Rd=1e-20}
      mask prompts: Lf "Lf (H)"; Rf "Rf (Ohm)"; Lc "Lc (H)"; Rc "Rc (Ohm)"; Cf "Cf (F)"; Rd "Rd (Ohm)"
  PQ Calculation (dq-Frame) : SimplexPS/PQ Calculation (dq-Frame)  SystemSampleTime=-1  VariantActivationTime=update diagram  Latency=0  AutoFrameSizeCalculation=off
  Unit Delay : UnitDelay  SampleTime=-1  HasFrameUpgradeWarning=on
  Voltage Controller : Subsystem  mask{Ts=Ts, Wbase=Wbase, Cf=Cf*(Sbase/Vbase^2)/Wbase, Kg=0, Kp=w_v*Cf*(Sbase/Vbase^2)/Wbase, Ki=w_v*w_v/4*Cf*(Sbase/Vbase^2)/Wbase*20, xdmax=inf, xqmax=inf, Kcd=0}
      mask prompts: Ts "Sampling Time (s)"; Wbase "Base Angular Frequency (rad/s)"; Cf "Capacitance"; Kg "Estimator Gain"; Kp "Proportional Gain"; Ki "Integral Gain"; xdmax "Current D Limit"; xqmax "Current Q Limit"; Kcd "Cross Decoupling Gain"
  "abc -> dq (Power-Invariant)" : SimplexPS/abc -> dq (Power-Invariant)  SystemSampleTime=-1  VariantActivationTime=update diagram  Latency=0  AutoFrameSizeCalculation=off
  "abc -> dq (Power-Invariant)1" : SimplexPS/abc -> dq (Power-Invariant)  SystemSampleTime=-1  VariantActivationTime=update diagram  Latency=0  AutoFrameSizeCalculation=off
  "abc -> dq (Power-Invariant)2" : SimplexPS/abc -> dq (Power-Invariant)  SystemSampleTime=-1  VariantActivationTime=update diagram  Latency=0  AutoFrameSizeCalculation=off
  "dq -> abc (Power-Invariant)" : SimplexPS/dq -> abc (Power-Invariant)  SystemSampleTime=-1  VariantActivationTime=update diagram  Latency=0  AutoFrameSizeCalculation=off
  va : powerlib/Electrical Sources/Controlled Voltage Source  Initialize=on  Source_Type=AC  Amplitude=0  Phase=0  Frequency=0  Measurements=None
  vb : powerlib/Electrical Sources/Controlled Voltage Source  Initialize=on  Source_Type=AC  Amplitude=0  Phase=0  Frequency=0  Measurements=None
  vc : powerlib/Electrical Sources/Controlled Voltage Source  Initialize=on  Source_Type=AC  Amplitude=0  Phase=0  Frequency=0  Measurements=None
  a : PMIOPort  Side=Right
  b : PMIOPort  Port=2  Side=Right
  c : PMIOPort  Port=3  Side=Right
  N : PMIOPort  Port=4  Side=Right
  m : Outport
  wires:
  [ig_dq] -> Voltage Controller/3(igdq)
  [vc_dq] -> Voltage Controller/2(vcdq)
  Constant1/1 -> Voltage Controller/4(enable)
  Voltage Controller/1(ildq*) -> Current Controller/1(iIdq*)
  vcdq*/1 -> Voltage Controller/1(vcdq*)
  [ig_abc] -> Bus Creator3/11  "igabc"
  [il_abc] -> Bus Creator3/10  "ilabc"
  [vc_abc] -> Bus Creator3/9  "vcabc"
  [vi_abc] -> Bus Creator3/8  "viabc"
  [ig_dq] -> Bus Creator3/7  "igdq"
  [il_dq] -> Bus Creator3/6  "ildq"
  [vc_dq] -> Bus Creator3/5  "vcdq"
  [vi_dq] -> Bus Creator3/4  "vidq"
  Gain1/1 -> Bus Creator3/3  "pq"
  [theta] -> Bus Creator3/2  "theta"
  Gain/1 -> Bus Creator3/1  "w"
  [pq] -> Gain1/1  "pq"
  [w] -> Gain/1  "w"
  Bus Selector/1 -> [vc_abc]  "<vcabc>"
  Unit Delay/1 -> Demux/1
  [vi_abc] -> Unit Delay/1
  [m_filter] -> Bus Selector/1
  "abc -> dq (Power-Invariant)1"/1 -> [il_dq]
  "abc -> dq (Power-Invariant)2"/1 -> [ig_dq]
  "abc -> dq (Power-Invariant)"/1 -> [vc_dq]
  [ig_abc] -> "Frequency Droop (iabc -> id)"/1
  [il_dq] -> Current Controller/2(iIdq)
  [ig_dq] -> PQ Calculation (dq-Frame)/2
  PQ Calculation (dq-Frame)/1 -> [pq]
  [vc_dq] -> PQ Calculation (dq-Frame)/1
  [theta] -> "dq -> abc (Power-Invariant)"/2
  Current Controller/1(vidq*) -> "dq -> abc (Power-Invariant)"/1, [vi_dq]
  [vc_dq] -> Current Controller/3(vdq)
  Constant/1 -> Current Controller/4(enable)
  "Frequency Droop (iabc -> id)"/1 -> [w]
  "Frequency Droop (iabc -> id)"/2 -> [theta]
  Bus Selector/2 -> [il_abc]  "<ilabc>"
  Bus Selector/3 -> [ig_abc]  "<igabc>"
  [theta] -> "abc -> dq (Power-Invariant)2"/2
  [ig_abc] -> "abc -> dq (Power-Invariant)2"/1
  [il_abc] -> "abc -> dq (Power-Invariant)1"/1
  [vc_abc] -> "abc -> dq (Power-Invariant)"/1
  [theta] -> "abc -> dq (Power-Invariant)1"/2
  [theta] -> "abc -> dq (Power-Invariant)"/2
  Demux/3 -> vc/1
  Demux/2 -> vb/1
  Demux/1 -> va/1
  LCL Filter/1(m) -> [m_filter]
  Bus Creator3/1 -> m/1
  "dq -> abc (Power-Invariant)"/1 -> [vi_abc]
  connections:
  LCL Filter/LConn3 -- vc/RConn1
  va/LConn1 -- vb/LConn1 -- vc/LConn1 -- LCL Filter/LConn4 -- N/RConn1
  LCL Filter/RConn3 -- c/RConn1
  LCL Filter/RConn2 -- b/RConn1
  LCL Filter/RConn1 -- a/RConn1
  LCL Filter/LConn1 -- va/RConn1
  LCL Filter/LConn2 -- vb/RConn1

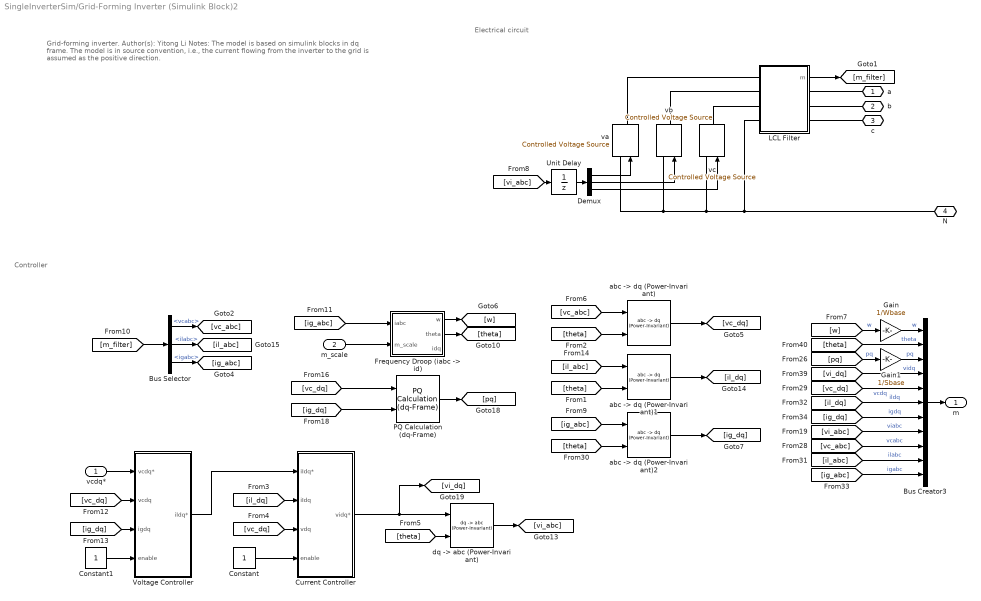
== system SingleInverterSim/Grid-Forming Inverter (Simulink Block)2 ==
  note: Grid-forming inverter.
      |
      | Author(s): Yitong Li
      |
      | Notes:
      |
      | The model is based on simulink blocks in dq frame.
      |
      | The model is in source convention, i.e., the current flowing from the inverter to the grid is assumed as the positive direction.
  note: Electrical circuit
  note: Controller
  vcdq* : Inport
  m_scale : Inport  Port=2
  Bus Creator3 : BusCreator  Inputs=11
  Bus Selector : BusSelector  OutputSignals=vcabc,ilabc,igabc
  Constant : Constant
  Constant1 : Constant
  Current Controller : Subsystem  mask{Ts=Ts, Wbase=Wbase, Lf=Lf*(Vbase^2/Sbase)/Wbase, Kg=0, Kp=w_i*Lf*(Vbase^2/Sbase)/Wbase, Ki=w_i*w_i/4*Lf*(Vbase^2/Sbase)/Wbase, xdmax=inf, xqmax=inf, Kcd=0}
      mask prompts: Ts "Sampling Time (s)"; Wbase "Base Angular Frequency (rad/s)"; Lf "Inductance"; Kg "Estimator Gain"; Kp "Proportional Gain"; Ki "Integral Gain"; xdmax "Voltage D Limit"; xqmax "Voltage Q Limit"; Kcd "Cross Decoupling Gain"
  Demux : Demux  Outputs=3
  "Frequency Droop (iabc -> id)" : Subsystem  AncestorBlock=|  mask{Ts=Ts, Sbase=Sbase, Vbase=Vbase, Wbase=Wbase, m=m, w_tau=w_droop, theta0=0, i0=0, w0=1}
      | SimplexPS/Frequency Droop
      | (iabc -> id)
      mask prompts: Ts "Ts (s), samping period"; Sbase "Sbase (VA), base power"; Vbase "Vbase (V), base voltage"; Wbase "Wbase (rad/s), base angular frequency"; m "m (pu), droop gain"; w_tau "w_tau (rad/s), low-pass filter bandwidth"; theta0 "theta0 (rad), initial angle"; i0 "i0 (pu), current setting point"; w0 "w0 (pu), frequency setting point"
  Gain : Gain  Gain=1/Wbase
  Gain1 : Gain  Gain=1/Sbase
  LCL Filter : Subsystem  AncestorBlock=SimplexPS/LCL Filter  mask{Lf=Lf*(Vbase^2/Sbase)/Wbase, Rf=Lf/10, Lc=Lc*(Vbase^2/Sbase)/Wbase, Rc=1e-20, Cf=Cf*(Sbase/Vbase^2)/Wbase, Rd=1e-20}
      mask prompts: Lf "Lf (H)"; Rf "Rf (Ohm)"; Lc "Lc (H)"; Rc "Rc (Ohm)"; Cf "Cf (F)"; Rd "Rd (Ohm)"
  PQ Calculation (dq-Frame) : SimplexPS/PQ Calculation (dq-Frame)  SystemSampleTime=-1  VariantActivationTime=update diagram  Latency=0  AutoFrameSizeCalculation=off
      settings: SourceProductName=Simplex Power Systems
  Unit Delay : UnitDelay  SampleTime=-1  HasFrameUpgradeWarning=on
  Voltage Controller : Subsystem  mask{Ts=Ts, Wbase=Wbase, Cf=Cf*(Sbase/Vbase^2)/Wbase, Kg=0, Kp=w_v*Cf*(Sbase/Vbase^2)/Wbase, Ki=w_v*w_v/4*Cf*(Sbase/Vbase^2)/Wbase*20, xdmax=inf, xqmax=inf, Kcd=0}
      mask prompts: Ts "Sampling Time (s)"; Wbase "Base Angular Frequency (rad/s)"; Cf "Capacitance"; Kg "Estimator Gain"; Kp "Proportional Gain"; Ki "Integral Gain"; xdmax "Current D Limit"; xqmax "Current Q Limit"; Kcd "Cross Decoupling Gain"
  "abc -> dq (Power-Invariant)" : SimplexPS/abc -> dq (Power-Invariant)  SystemSampleTime=-1  VariantActivationTime=update diagram  Latency=0  AutoFrameSizeCalculation=off
      settings: SourceProductName=Simplex Power Systems
  "abc -> dq (Power-Invariant)1" : SimplexPS/abc -> dq (Power-Invariant)  SystemSampleTime=-1  VariantActivationTime=update diagram  Latency=0  AutoFrameSizeCalculation=off
      settings: SourceProductName=Simplex Power Systems
  "abc -> dq (Power-Invariant)2" : SimplexPS/abc -> dq (Power-Invariant)  SystemSampleTime=-1  VariantActivationTime=update diagram  Latency=0  AutoFrameSizeCalculation=off
      settings: SourceProductName=Simplex Power Systems
  "dq -> abc (Power-Invariant)" : SimplexPS/dq -> abc (Power-Invariant)  SystemSampleTime=-1  VariantActivationTime=update diagram  Latency=0  AutoFrameSizeCalculation=off
      settings: SourceProductName=Simplex Power Systems
  va : powerlib/Electrical Sources/Controlled Voltage Source  Initialize=on  Source_Type=AC  Amplitude=0  Phase=0  Frequency=0  Measurements=None
  vb : powerlib/Electrical Sources/Controlled Voltage Source  Initialize=on  Source_Type=AC  Amplitude=0  Phase=0  Frequency=0  Measurements=None
  vc : powerlib/Electrical Sources/Controlled Voltage Source  Initialize=on  Source_Type=AC  Amplitude=0  Phase=0  Frequency=0  Measurements=None
  a : PMIOPort  Side=Right
  b : PMIOPort  Port=2  Side=Right
  c : PMIOPort  Port=3  Side=Right
  N : PMIOPort  Port=4  Side=Right
  m : Outport
  wires:
  [ig_dq] -> Voltage Controller/3(igdq)
  [vc_dq] -> Voltage Controller/2(vcdq)
  Constant1/1 -> Voltage Controller/4(enable)
  Voltage Controller/1(ildq*) -> Current Controller/1(iIdq*)
  vcdq*/1 -> Voltage Controller/1(vcdq*)
  [ig_abc] -> Bus Creator3/11  "igabc"
  [il_abc] -> Bus Creator3/10  "ilabc"
  [vc_abc] -> Bus Creator3/9  "vcabc"
  [vi_abc] -> Bus Creator3/8  "viabc"
  [ig_dq] -> Bus Creator3/7  "igdq"
  [il_dq] -> Bus Creator3/6  "ildq"
  [vc_dq] -> Bus Creator3/5  "vcdq"
  [vi_dq] -> Bus Creator3/4  "vidq"
  Gain1/1 -> Bus Creator3/3  "pq"
  [theta] -> Bus Creator3/2  "theta"
  Gain/1 -> Bus Creator3/1  "w"
  [pq] -> Gain1/1  "pq"
  [w] -> Gain/1  "w"
  Bus Selector/1 -> [vc_abc]  "<vcabc>"
  Unit Delay/1 -> Demux/1
  [vi_abc] -> Unit Delay/1
  [m_filter] -> Bus Selector/1
  "abc -> dq (Power-Invariant)1"/1 -> [il_dq]
  "abc -> dq (Power-Invariant)2"/1 -> [ig_dq]
  "abc -> dq (Power-Invariant)"/1 -> [vc_dq]
  [ig_abc] -> "Frequency Droop (iabc -> id)"/1(iabc)
  [il_dq] -> Current Controller/2(iIdq)
  [ig_dq] -> PQ Calculation (dq-Frame)/2
  PQ Calculation (dq-Frame)/1 -> [pq]
  [vc_dq] -> PQ Calculation (dq-Frame)/1
  [theta] -> "dq -> abc (Power-Invariant)"/2
  Current Controller/1(vidq*) -> "dq -> abc (Power-Invariant)"/1, [vi_dq]
  [vc_dq] -> Current Controller/3(vdq)
  Constant/1 -> Current Controller/4(enable)
  "Frequency Droop (iabc -> id)"/1(w) -> [w]
  "Frequency Droop (iabc -> id)"/2(theta) -> [theta]
  Bus Selector/2 -> [il_abc]  "<ilabc>"
  Bus Selector/3 -> [ig_abc]  "<igabc>"
  [theta] -> "abc -> dq (Power-Invariant)2"/2
  [ig_abc] -> "abc -> dq (Power-Invariant)2"/1
  [il_abc] -> "abc -> dq (Power-Invariant)1"/1
  [vc_abc] -> "abc -> dq (Power-Invariant)"/1
  [theta] -> "abc -> dq (Power-Invariant)1"/2
  [theta] -> "abc -> dq (Power-Invariant)"/2
  Demux/3 -> vc/1
  Demux/2 -> vb/1
  Demux/1 -> va/1
  LCL Filter/1(m) -> [m_filter]
  Bus Creator3/1 -> m/1
  "dq -> abc (Power-Invariant)"/1 -> [vi_abc]
  m_scale/1 -> "Frequency Droop (iabc -> id)"/2(m_scale)
  connections:
  LCL Filter/LConn3 -- vc/RConn1
  va/LConn1 -- vb/LConn1 -- vc/LConn1 -- LCL Filter/LConn4 -- N/RConn1
  LCL Filter/RConn3 -- c/RConn1
  LCL Filter/RConn2 -- b/RConn1
  LCL Filter/RConn1 -- a/RConn1
  LCL Filter/LConn1 -- va/RConn1
  LCL Filter/LConn2 -- vb/RConn1

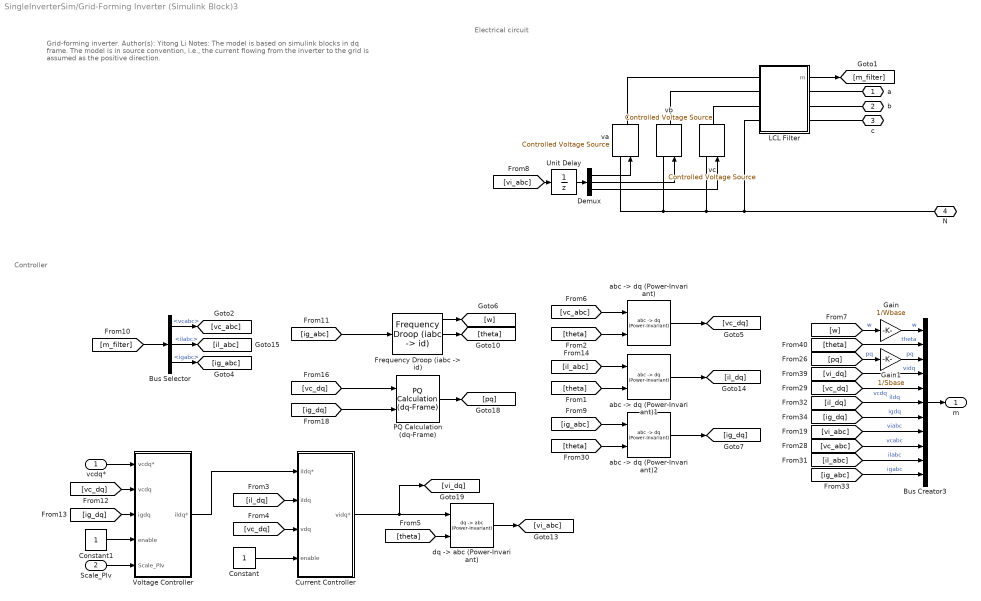
== system SingleInverterSim/Grid-Forming Inverter (Simulink Block)3 ==
  note: Grid-forming inverter.
      |
      | Author(s): Yitong Li
      |
      | Notes:
      |
      | The model is based on simulink blocks in dq frame.
      |
      | The model is in source convention, i.e., the current flowing from the inverter to the grid is assumed as the positive direction.
  note: Electrical circuit
  note: Controller
  vcdq* : Inport
  Scale_PIv : Inport  Port=2
  Bus Creator3 : BusCreator  Inputs=11
  Bus Selector : BusSelector  OutputSignals=vcabc,ilabc,igabc
  Constant : Constant
  Constant1 : Constant
  Current Controller : Subsystem  mask{Ts=Ts, Wbase=Wbase, Lf=Lf*(Vbase^2/Sbase)/Wbase, Kg=0, Kp=w_i*Lf*(Vbase^2/Sbase)/Wbase, Ki=w_i*w_i/4*Lf*(Vbase^2/Sbase)/Wbase, xdmax=inf, xqmax=inf, Kcd=0}
      mask prompts: Ts "Sampling Time (s)"; Wbase "Base Angular Frequency (rad/s)"; Lf "Inductance"; Kg "Estimator Gain"; Kp "Proportional Gain"; Ki "Integral Gain"; xdmax "Voltage D Limit"; xqmax "Voltage Q Limit"; Kcd "Cross Decoupling Gain"
  Demux : Demux  Outputs=3
  "Frequency Droop (iabc -> id)" : SimplexPS/Frequency Droop (iabc -> id)  Ts=Ts  Sbase=Sbase  Vbase=Vbase  Wbase=Wbase  m=m  w_tau=w_droop  theta0=0  i0=0  w0=1
      settings: SourceProductName=Simplex Power Systems
  Gain : Gain  Gain=1/Wbase
  Gain1 : Gain  Gain=1/Sbase
  LCL Filter : Subsystem  AncestorBlock=SimplexPS/LCL Filter  mask{Lf=Lf*(Vbase^2/Sbase)/Wbase, Rf=Lf/10, Lc=Lc*(Vbase^2/Sbase)/Wbase, Rc=1e-20, Cf=Cf*(Sbase/Vbase^2)/Wbase, Rd=1e-20}
      mask prompts: Lf "Lf (H)"; Rf "Rf (Ohm)"; Lc "Lc (H)"; Rc "Rc (Ohm)"; Cf "Cf (F)"; Rd "Rd (Ohm)"
  PQ Calculation (dq-Frame) : SimplexPS/PQ Calculation (dq-Frame)  SystemSampleTime=-1  VariantActivationTime=update diagram  Latency=0  AutoFrameSizeCalculation=off
      settings: SourceProductName=Simplex Power Systems
  Unit Delay : UnitDelay  SampleTime=-1  HasFrameUpgradeWarning=on
  Voltage Controller : Subsystem  mask{Ts=Ts, Wbase=Wbase, Cf=Cf*(Sbase/Vbase^2)/Wbase, Kg=0, Kp=w_v*Cf*(Sbase/Vbase^2)/Wbase, Ki=w_v*w_v/4*Cf*(Sbase/Vbase^2)/Wbase*20, xdmax=inf, xqmax=inf, Kcd=0}
      mask prompts: Ts "Sampling Time (s)"; Wbase "Base Angular Frequency (rad/s)"; Cf "Capacitance"; Kg "Estimator Gain"; Kp "Proportional Gain"; Ki "Integral Gain"; xdmax "Current D Limit"; xqmax "Current Q Limit"; Kcd "Cross Decoupling Gain"
  "abc -> dq (Power-Invariant)" : SimplexPS/abc -> dq (Power-Invariant)  SystemSampleTime=-1  VariantActivationTime=update diagram  Latency=0  AutoFrameSizeCalculation=off
      settings: SourceProductName=Simplex Power Systems
  "abc -> dq (Power-Invariant)1" : SimplexPS/abc -> dq (Power-Invariant)  SystemSampleTime=-1  VariantActivationTime=update diagram  Latency=0  AutoFrameSizeCalculation=off
      settings: SourceProductName=Simplex Power Systems
  "abc -> dq (Power-Invariant)2" : SimplexPS/abc -> dq (Power-Invariant)  SystemSampleTime=-1  VariantActivationTime=update diagram  Latency=0  AutoFrameSizeCalculation=off
      settings: SourceProductName=Simplex Power Systems
  "dq -> abc (Power-Invariant)" : SimplexPS/dq -> abc (Power-Invariant)  SystemSampleTime=-1  VariantActivationTime=update diagram  Latency=0  AutoFrameSizeCalculation=off
      settings: SourceProductName=Simplex Power Systems
  va : powerlib/Electrical Sources/Controlled Voltage Source  Initialize=on  Source_Type=AC  Amplitude=0  Phase=0  Frequency=0  Measurements=None
  vb : powerlib/Electrical Sources/Controlled Voltage Source  Initialize=on  Source_Type=AC  Amplitude=0  Phase=0  Frequency=0  Measurements=None
  vc : powerlib/Electrical Sources/Controlled Voltage Source  Initialize=on  Source_Type=AC  Amplitude=0  Phase=0  Frequency=0  Measurements=None
  a : PMIOPort  Side=Right
  b : PMIOPort  Port=2  Side=Right
  c : PMIOPort  Port=3  Side=Right
  N : PMIOPort  Port=4  Side=Right
  m : Outport
  wires:
  [ig_dq] -> Voltage Controller/3(igdq)
  [vc_dq] -> Voltage Controller/2(vcdq)
  Constant1/1 -> Voltage Controller/4(enable)
  Voltage Controller/1(ildq*) -> Current Controller/1(iIdq*)
  vcdq*/1 -> Voltage Controller/1(vcdq*)
  [ig_abc] -> Bus Creator3/11  "igabc"
  [il_abc] -> Bus Creator3/10  "ilabc"
  [vc_abc] -> Bus Creator3/9  "vcabc"
  [vi_abc] -> Bus Creator3/8  "viabc"
  [ig_dq] -> Bus Creator3/7  "igdq"
  [il_dq] -> Bus Creator3/6  "ildq"
  [vc_dq] -> Bus Creator3/5  "vcdq"
  [vi_dq] -> Bus Creator3/4  "vidq"
  Gain1/1 -> Bus Creator3/3  "pq"
  [theta] -> Bus Creator3/2  "theta"
  Gain/1 -> Bus Creator3/1  "w"
  [pq] -> Gain1/1  "pq"
  [w] -> Gain/1  "w"
  Bus Selector/1 -> [vc_abc]  "<vcabc>"
  Unit Delay/1 -> Demux/1
  [vi_abc] -> Unit Delay/1
  [m_filter] -> Bus Selector/1
  "abc -> dq (Power-Invariant)1"/1 -> [il_dq]
  "abc -> dq (Power-Invariant)2"/1 -> [ig_dq]
  "abc -> dq (Power-Invariant)"/1 -> [vc_dq]
  [ig_abc] -> "Frequency Droop (iabc -> id)"/1
  [il_dq] -> Current Controller/2(iIdq)
  [ig_dq] -> PQ Calculation (dq-Frame)/2
  PQ Calculation (dq-Frame)/1 -> [pq]
  [vc_dq] -> PQ Calculation (dq-Frame)/1
  [theta] -> "dq -> abc (Power-Invariant)"/2
  Current Controller/1(vidq*) -> "dq -> abc (Power-Invariant)"/1, [vi_dq]
  [vc_dq] -> Current Controller/3(vdq)
  Constant/1 -> Current Controller/4(enable)
  "Frequency Droop (iabc -> id)"/1 -> [w]
  "Frequency Droop (iabc -> id)"/2 -> [theta]
  Bus Selector/2 -> [il_abc]  "<ilabc>"
  Bus Selector/3 -> [ig_abc]  "<igabc>"
  [theta] -> "abc -> dq (Power-Invariant)2"/2
  [ig_abc] -> "abc -> dq (Power-Invariant)2"/1
  [il_abc] -> "abc -> dq (Power-Invariant)1"/1
  [vc_abc] -> "abc -> dq (Power-Invariant)"/1
  [theta] -> "abc -> dq (Power-Invariant)1"/2
  [theta] -> "abc -> dq (Power-Invariant)"/2
  Demux/3 -> vc/1
  Demux/2 -> vb/1
  Demux/1 -> va/1
  LCL Filter/1(m) -> [m_filter]
  Bus Creator3/1 -> m/1
  "dq -> abc (Power-Invariant)"/1 -> [vi_abc]
  Scale_PIv/1 -> Voltage Controller/5(Scale_PIv)
  connections:
  LCL Filter/LConn3 -- vc/RConn1
  va/LConn1 -- vb/LConn1 -- vc/LConn1 -- LCL Filter/LConn4 -- N/RConn1
  LCL Filter/RConn3 -- c/RConn1
  LCL Filter/RConn2 -- b/RConn1
  LCL Filter/RConn1 -- a/RConn1
  LCL Filter/LConn1 -- va/RConn1
  LCL Filter/LConn2 -- vb/RConn1
